simulink library "halout"  (R2021b)
settings: Solver=VariableStepAuto  StartTime=0.0  StopTime=10.0  RelTol=1e-3
undefined symbols (not defined in the file): C_TASK_5MS_S, FALSE, KHAL_CAN1FD1APS3E2E_flg, KHAL_CAN1FD1APS3TxReq_flg, KHAL_CAN1FD1VCU2E2E_flg, KHAL_CAN1FD1VCU2TxReq_flg, KHAL_CAN1FD1VCU3E2E_flg, KHAL_CAN1FD1VCU3TxReq_flg, KHAL_CAN1TxReq_flg, KHAL_CAN1VMCFCM1E2E_flg, KHAL_CAN1VMCFCM1TxReq_flg, KHAL_CAN2TxReq_flg, KHAL_CAN3FD3VCU1toNIDECTxReq_flg, KHAL_CAN3FD3VCU1TxReq_flg, KHAL_CAN3FD3VCU2E2E_flg, KHAL_CAN3FD3VCU2toNIDECE2E_flg, KHAL_CAN3FD3VCU2toNIDECTxReq_flg, KHAL_CAN3FD3VCU2TxReq_flg, KHAL_CAN3TxReq_flg, KHAL_CAN4FD4CE1000E2E_flg, KHAL_CAN4FD4CE1000TxReq_flg, KHAL_CAN4TxReq_flg, KHAL_CAN5TxReq_flg, KHAL_CAN6FD6APS3E2E_flg, KHAL_CAN6FD6APS3TxReq_flg, KHAL_CAN6FD6VCU2E2E_flg, KHAL_CAN6FD6VCU2TxReq_flg, KHAL_CAN6TxReq_flg, ONE_INT, TRUE, ZERO_INT
libraries: FVT_lib x549, simulink x244
(part 7 of 27)

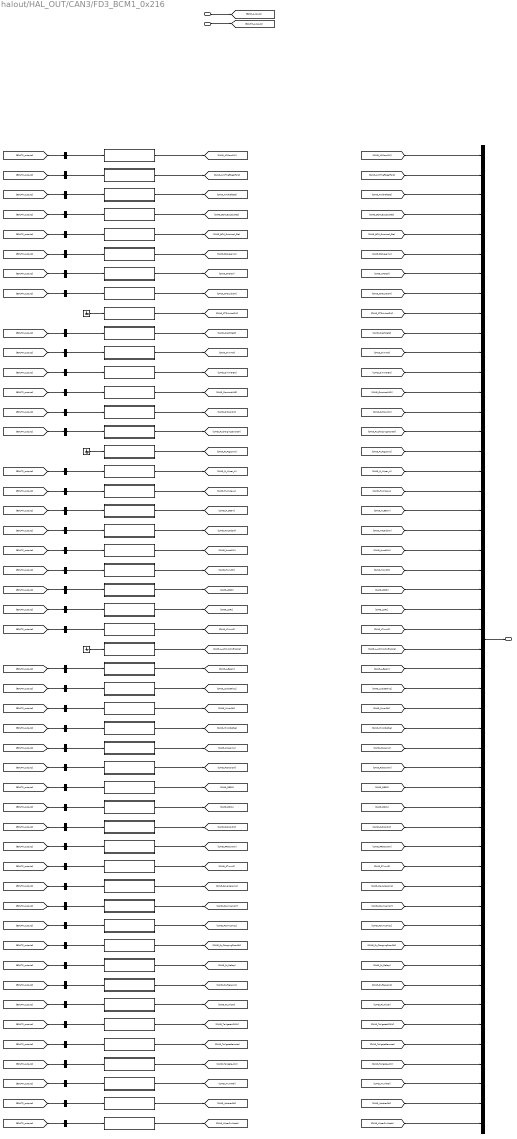
== system halout/HAL_OUT/CAN3/FD3_BCM1_0x216 ==
  BSCP_outputs : Inport  OutDataTypeStr=Bus: BSCP_outputs
  BOUTP_outputs : Inport  Port=2  OutDataTypeStr=Bus: BOUTP_outputs
  AllDoorSW : Subsystem
  AntiTheftSeatFold : Subsystem
  AntitheftSta : Subsystem
  BCMBuzzerReq : Subsystem
  BCMDoorLockSta : Subsystem
  BrakeLamp : Subsystem
  CTDCtrl : Subsystem
  CTDLockSW : Subsystem
  CTDUnlockSW : Subsystem
  CrashDetd : Subsystem
  Dimmer : Subsystem
  DimmerEN : Subsystem
  DoorLockIND : Subsystem
  DrDoorSW : Subsystem
  FrChargingDoorCtrl : Subsystem
  FrFogLamp : Subsystem
  FrWiperH : Subsystem
  FrWiperL : Subsystem
  Ground : Ground
  Ground1 : Ground
  Ground2 : Ground
  HBeam : Subsystem
  HazardSW : Subsystem
  HoodSW : Subsystem
  HornCtrl : Subsystem
  LAPMWdwEnable : Subsystem
  LBSD : Subsystem
  LBeam : Subsystem
  LDRL : Subsystem
  LTurnLP : Subsystem
  LockSetting : Subsystem
  MirrorCtrl : Subsystem
  MirrorDefog : Subsystem
  PosLamp : Subsystem
  PsDoorSW : Subsystem
  RBSD : Subsystem
  RDRL : Subsystem
  RLDoorSW : Subsystem
  RRDoorSW : Subsystem
  RTurnLP : Subsystem
  ReverseLamp : Subsystem
  RoomLampH : Subsystem
  RoomLampL : Subsystem
  RrChargingDoorCtrl : Subsystem
  RrDefog : Subsystem
  RrFogLamp : Subsystem
  RrWiper : Subsystem
  TailgateHDSW : Subsystem
  TailgateRemote : Subsystem
  TailgateSW : Subsystem
  TrunkRel : Subsystem
  WasherCtrl : Subsystem
  WiperFixMode : Subsystem
  bus_creator : BusCreator  Inputs=50  OutDataTypeStr=Bus: DT_CAN3_SG_FD3_BCM1  NonVirtualBus=on
  bus_selector : BusSelector  OutputSignals=VOUTP_AllDoorSW_flg
  bus_selector1 : BusSelector  OutputSignals=VOUTP_AntitheftSeatFlod_flg
  bus_selector10 : BusSelector  OutputSignals=VOUTP_DimmerEN_flg
  bus_selector11 : BusSelector  OutputSignals=VOUTP_DoorLockIND_flg
  bus_selector12 : BusSelector  OutputSignals=VOUTP_DrDoorSW_flg
  bus_selector13 : BusSelector  OutputSignals=VOUTP_FrChargingDoorCtrl_enum
  bus_selector14 : BusSelector  OutputSignals=VOUTP_FrWiperH_flg
  bus_selector15 : BusSelector  OutputSignals=VOUTP_FrWiperL_flg
  bus_selector16 : BusSelector  OutputSignals=VOUTP_HBeam_flg
  bus_selector17 : BusSelector  OutputSignals=VOUTP_HazardSW_flg
  bus_selector18 : BusSelector  OutputSignals=VOUTP_HoodSW_flg
  bus_selector19 : BusSelector  OutputSignals=VOUTP_HornCtrl_flg
  bus_selector2 : BusSelector  OutputSignals=VOUTP_AntitheftSta_enum
  bus_selector20 : BusSelector  OutputSignals=VOUTP_LBSD_flg
  bus_selector21 : BusSelector  OutputSignals=VOUTP_LDRL_flg
  bus_selector22 : BusSelector  OutputSignals=VOUTP_LTurnLP_flg
  bus_selector23 : BusSelector  OutputSignals=VOUTP_LBeam_flg
  bus_selector24 : BusSelector  OutputSignals=VOUTP_LockSetting_flg
  bus_selector25 : BusSelector  OutputSignals=VOUTP_MirrorCtrl_enum
  bus_selector26 : BusSelector  OutputSignals=VOUTP_MirrorDefog_flg
  bus_selector27 : BusSelector  OutputSignals=VOUTP_PosLamp_flg
  bus_selector28 : BusSelector  OutputSignals=VOUTP_PsDoorSW_flg
  bus_selector29 : BusSelector  OutputSignals=VOUTP_RBSD_flg
  bus_selector3 : BusSelector  OutputSignals=VOUTP_BCMBuzzerReq_flg
  bus_selector30 : BusSelector  OutputSignals=VOUTP_RDRL_flg
  bus_selector31 : BusSelector  OutputSignals=VOUTP_RLDoorSW_flg
  bus_selector32 : BusSelector  OutputSignals=VOUTP_RRDoorSW_flg
  bus_selector33 : BusSelector  OutputSignals=VOUTP_RTurnLP_flg
  bus_selector34 : BusSelector  OutputSignals=VOUTP_ReverseLamp_flg
  bus_selector35 : BusSelector  OutputSignals=VOUTP_RoomLampH_flg
  bus_selector36 : BusSelector  OutputSignals=VOUTP_RoomLampL_flg
  bus_selector37 : BusSelector  OutputSignals=VOUTP_RrChargingDoorCtrl_enum
  bus_selector38 : BusSelector  OutputSignals=VOUTP_RrDefog_flg
  bus_selector39 : BusSelector  OutputSignals=VOUTP_RrFogLamp_flg
  bus_selector4 : BusSelector  OutputSignals=VOUTP_BCMDoorLockSta_flg
  bus_selector40 : BusSelector  OutputSignals=VOUTP_RrWiper_flg
  bus_selector41 : BusSelector  OutputSignals=VOUTP_TailgateHDSW_flg
  bus_selector42 : BusSelector  OutputSignals=VOUTP_TailgateRemote_enum
  bus_selector43 : BusSelector  OutputSignals=VOUTP_TailgateSW_flg
  bus_selector44 : BusSelector  OutputSignals=VOUTP_TrunkRel_flg
  bus_selector45 : BusSelector  OutputSignals=VOUTP_WasherCtrl_enum
  bus_selector46 : BusSelector  OutputSignals=VOUTP_WiperFixMode_flg
  bus_selector5 : BusSelector  OutputSignals=VOUTP_BrakeLamp_flg
  bus_selector6 : BusSelector  OutputSignals=VOUTP_CTDCtrl_enum
  bus_selector7 : BusSelector  OutputSignals=VOUTP_CTDLockSW_flg
  bus_selector8 : BusSelector  OutputSignals=VOUTP_CrashDetd_flg
  bus_selector9 : BusSelector  OutputSignals=VOUTP_Dimmer_pct
  FD3_BCM1 : Outport
  wires:
  BSCP_outputs/1 -> [BSCP_outputs]
  BOUTP_outputs/1 -> [BOUTP_outputs]
  [CAN3_AllDoorSW] -> bus_creator/1  "CAN3_AllDoorSW"
  [CAN3_AntiTheftSeatFold] -> bus_creator/2  "CAN3_AntiTheftSeatFold"
  [CAN3_AntitheftSta] -> bus_creator/3  "CAN3_AntitheftSta"
  [CAN3_BCM_Buzzer_Req] -> bus_creator/4  "CAN3_BCM_Buzzer_Req"
  [CAN3_BCM_DoorLock_Sta] -> bus_creator/5  "CAN3_BCM_DoorLock_Sta"
  [CAN3_BrakeLamp] -> bus_creator/6  "CAN3_BrakeLamp"
  [CAN3_CTDCtrl] -> bus_creator/7  "CAN3_CTDCtrl"
  [CAN3_CTDLockSW] -> bus_creator/8  "CAN3_CTDLockSW"
  [CAN3_CTDUnlockSW] -> bus_creator/9  "CAN3_CTDUnlockSW"
  [CAN3_CrashDetd] -> bus_creator/10  "CAN3_CrashDetd"
  [CAN3_Dimmer] -> bus_creator/11  "CAN3_Dimmer"
  [CAN3_DimmerEN] -> bus_creator/12  "CAN3_DimmerEN"
  [CAN3_DoorLockIND] -> bus_creator/13  "CAN3_DoorLockIND"
  [CAN3_DrDoorSW] -> bus_creator/14  "CAN3_DrDoorSW"
  [CAN3_Fr_ChargingDoorCtrl] -> bus_creator/15  "CAN3_Fr_ChargingDoorCtrl"
  [CAN3_Fr_FogLamp] -> bus_creator/16  "CAN3_Fr_FogLamp"
  [CAN3_Fr_Wiper_H] -> bus_creator/17  "CAN3_Fr_Wiper_H"
  [CAN3_Fr_Wiper_L] -> bus_creator/18  "CAN3_Fr_Wiper_L"
  [CAN3_H_Beam] -> bus_creator/19  "CAN3_H_Beam"
  [CAN3_HazardSW] -> bus_creator/20  "CAN3_HazardSW"
  [CAN3_HoodSW] -> bus_creator/21  "CAN3_HoodSW"
  [CAN3_HornCtrl] -> bus_creator/22  "CAN3_HornCtrl"
  [CAN3_LBSD] -> bus_creator/23  "CAN3_LBSD"
  [CAN3_LDRL] -> bus_creator/24  "CAN3_LDRL"
  [CAN3_LTurnLP] -> bus_creator/25  "CAN3_LTurnLP"
  [CAN3_L_APM_WdwEnable] -> bus_creator/26  "CAN3_L_APM_WdwEnable"
  [CAN3_L_Beam] -> bus_creator/27  "CAN3_L_Beam"
  [CAN3_LockSetting] -> bus_creator/28  "CAN3_LockSetting"
  [CAN3_MirrorCtrl] -> bus_creator/29  "CAN3_MirrorCtrl"
  [CAN3_MirrorDefog] -> bus_creator/30  "CAN3_MirrorDefog"
  [CAN3_PosLamp] -> bus_creator/31  "CAN3_PosLamp"
  [CAN3_PsDoorSW] -> bus_creator/32  "CAN3_PsDoorSW"
  [CAN3_RBSD] -> bus_creator/33  "CAN3_RBSD"
  [CAN3_RDRL] -> bus_creator/34  "CAN3_RDRL"
  [CAN3_RLDoorSW] -> bus_creator/35  "CAN3_RLDoorSW"
  [CAN3_RRDoorSW] -> bus_creator/36  "CAN3_RRDoorSW"
  [CAN3_RTurnLP] -> bus_creator/37  "CAN3_RTurnLP"
  [CAN3_ReverseLamp] -> bus_creator/38  "CAN3_ReverseLamp"
  [CAN3_RoomLampH] -> bus_creator/39  "CAN3_RoomLampH"
  [CAN3_RoomLampL] -> bus_creator/40  "CAN3_RoomLampL"
  [CAN3_Rr_ChargingDoorCtrl] -> bus_creator/41  "CAN3_Rr_ChargingDoorCtrl"
  [CAN3_Rr_Defog] -> bus_creator/42  "CAN3_Rr_Defog"
  [CAN3_Rr_FogLamp] -> bus_creator/43  "CAN3_Rr_FogLamp"
  [CAN3_Rr_Wiper] -> bus_creator/44  "CAN3_Rr_Wiper"
  [CAN3_TailgateHDSW] -> bus_creator/45  "CAN3_TailgateHDSW"
  [CAN3_TailgateRemote] -> bus_creator/46  "CAN3_TailgateRemote"
  [CAN3_Tailgate_SW] -> bus_creator/47  "CAN3_Tailgate_SW"
  [CAN3_TrunkRel] -> bus_creator/48  "CAN3_TrunkRel"
  [CAN3_WasherCtrl] -> bus_creator/49  "CAN3_WasherCtrl"
  [CAN3_WiperFixMode] -> bus_creator/50  "CAN3_WiperFixMode"
  bus_creator/1 -> FD3_BCM1/1
  AllDoorSW/1(CAN3_AllDoorSW) -> [CAN3_AllDoorSW]
  AntiTheftSeatFold/1(CAN3_AntiTheftSeatFold) -> [CAN3_AntiTheftSeatFold]
  AntitheftSta/1(CAN3_AntitheftSta) -> [CAN3_AntitheftSta]
  BCMBuzzerReq/1(CAN3_BCM_Buzzer_Req) -> [CAN3_BCM_Buzzer_Req]
  BCMDoorLockSta/1(CAN3_BCM_DoorLock_Sta) -> [CAN3_BCM_DoorLock_Sta]
  BrakeLamp/1(CAN3_BrakeLamp) -> [CAN3_BrakeLamp]
  CTDCtrl/1(CAN3_CTDCtrl) -> [CAN3_CTDCtrl]
  CTDLockSW/1(CAN3_CTDLockSW) -> [CAN3_CTDLockSW]
  CTDUnlockSW/1(CAN3_CTDUnlockSW) -> [CAN3_CTDUnlockSW]
  CrashDetd/1(CAN3_CrashDetd) -> [CAN3_CrashDetd]
  Dimmer/1(CAN3_Dimmer) -> [CAN3_Dimmer]
  DimmerEN/1(CAN3_DimmerEN) -> [CAN3_DimmerEN]
  DoorLockIND/1(CAN3_DoorLockIND) -> [CAN3_DoorLockIND]
  DrDoorSW/1(CAN3_DrDoorSW) -> [CAN3_DrDoorSW]
  FrChargingDoorCtrl/1(CAN3_Fr_ChargingDoorCtrl) -> [CAN3_Fr_ChargingDoorCtrl]
  FrFogLamp/1(CAN3_Fr_FogLamp) -> [CAN3_Fr_FogLamp]
  FrWiperH/1(CAN3_Fr_Wiper_H) -> [CAN3_Fr_Wiper_H]
  FrWiperL/1(CAN3_Fr_Wiper_L) -> [CAN3_Fr_Wiper_L]
  HBeam/1(CAN3_H_Beam) -> [CAN3_H_Beam]
  HazardSW/1(CAN3_HazardSW) -> [CAN3_HazardSW]
  HoodSW/1(CAN3_HoodSW) -> [CAN3_HoodSW]
  HornCtrl/1(CAN3_HornCtrl) -> [CAN3_HornCtrl]
  LBSD/1(CAN3_LBSD) -> [CAN3_LBSD]
  LDRL/1(CAN3_LDRL) -> [CAN3_LDRL]
  LTurnLP/1(CAN3_LTurnLP) -> [CAN3_LTurnLP]
  LAPMWdwEnable/1(CAN3_L_APM_WdwEnable) -> [CAN3_L_APM_WdwEnable]
  LBeam/1(CAN3_L_Beam) -> [CAN3_L_Beam]
  LockSetting/1(CAN3_LockSetting) -> [CAN3_LockSetting]
  MirrorCtrl/1(CAN3_MirrorCtrl) -> [CAN3_MirrorCtrl]
  MirrorDefog/1(CAN3_MirrorDefog) -> [CAN3_MirrorDefog]
  PosLamp/1(CAN3_PosLamp) -> [CAN3_PosLamp]
  PsDoorSW/1(CAN3_PsDoorSW) -> [CAN3_PsDoorSW]
  RBSD/1(CAN3_RBSD) -> [CAN3_RBSD]
  RDRL/1(CAN3_RDRL) -> [CAN3_RDRL]
  RLDoorSW/1(CAN3_RLDoorSW) -> [CAN3_RLDoorSW]
  RRDoorSW/1(CAN3_RRDoorSW) -> [CAN3_RRDoorSW]
  RTurnLP/1(CAN3_RTurnLP) -> [CAN3_RTurnLP]
  ReverseLamp/1(CAN3_ReverseLamp) -> [CAN3_ReverseLamp]
  RoomLampH/1(CAN3_RoomLampH) -> [CAN3_RoomLampH]
  RoomLampL/1(CAN3_RoomLampL) -> [CAN3_RoomLampL]
  RrChargingDoorCtrl/1(CAN3_Rr_ChargingDoorCtrl) -> [CAN3_Rr_ChargingDoorCtrl]
  RrDefog/1(CAN3_Rr_Defog) -> [CAN3_Rr_Defog]
  RrFogLamp/1(CAN3_Rr_FogLamp) -> [CAN3_Rr_FogLamp]
  RrWiper/1(CAN3_Rr_Wiper) -> [CAN3_Rr_Wiper]
  TailgateHDSW/1(CAN3_TailgateHDSW) -> [CAN3_TailgateHDSW]
  TailgateRemote/1(CAN3_TailgateRemote) -> [CAN3_TailgateRemote]
  TailgateSW/1(CAN3_Tailgate_SW) -> [CAN3_Tailgate_SW]
  TrunkRel/1(CAN3_TrunkRel) -> [CAN3_TrunkRel]
  WasherCtrl/1(CAN3_WasherCtrl) -> [CAN3_WasherCtrl]
  WiperFixMode/1(CAN3_WiperFixMode) -> [CAN3_WiperFixMode]
  bus_selector/1 -> AllDoorSW/1(AllDoorSW)  "<VOUTP_AllDoorSW_flg>"
  [BOUTP_outputs] -> bus_selector/1
  bus_selector1/1 -> AntiTheftSeatFold/1(AntiTheftSeatFold)  "<VOUTP_AntitheftSeatFlod_flg>"
  [BOUTP_outputs] -> bus_selector1/1
  bus_selector2/1 -> AntitheftSta/1(AntitheftSta)  "<VOUTP_AntitheftSta_enum>"
  [BOUTP_outputs] -> bus_selector2/1
  bus_selector3/1 -> BCMBuzzerReq/1(BCMBuzzerReq)  "<VOUTP_BCMBuzzerReq_flg>"
  [BOUTP_outputs] -> bus_selector3/1
  bus_selector4/1 -> BCMDoorLockSta/1(BCMDoorLockSta)  "<VOUTP_BCMDoorLockSta_flg>"
  [BOUTP_outputs] -> bus_selector4/1
  bus_selector5/1 -> BrakeLamp/1(BrakeLamp)  "<VOUTP_BrakeLamp_flg>"
  [BOUTP_outputs] -> bus_selector5/1
  bus_selector6/1 -> CTDCtrl/1(CTDCtrl)  "<VOUTP_CTDCtrl_enum>"
  [BOUTP_outputs] -> bus_selector6/1
  bus_selector7/1 -> CTDLockSW/1(CTDLockSW)  "<VOUTP_CTDLockSW_flg>"
  [BOUTP_outputs] -> bus_selector7/1
  Ground/1 -> CTDUnlockSW/1(CTDUnlockSW)
  bus_selector8/1 -> CrashDetd/1(CrashDetd)  "<VOUTP_CrashDetd_flg>"
  [BOUTP_outputs] -> bus_selector8/1
  bus_selector9/1 -> Dimmer/1(Dimmer)  "<VOUTP_Dimmer_pct>"
  [BOUTP_outputs] -> bus_selector9/1
  bus_selector10/1 -> DimmerEN/1(DimmerEN)  "<VOUTP_DimmerEN_flg>"
  [BOUTP_outputs] -> bus_selector10/1
  bus_selector11/1 -> DoorLockIND/1(DoorLockIND)  "<VOUTP_DoorLockIND_flg>"
  [BOUTP_outputs] -> bus_selector11/1
  bus_selector12/1 -> DrDoorSW/1(DrDoorSW)  "<VOUTP_DrDoorSW_flg>"
  [BOUTP_outputs] -> bus_selector12/1
  bus_selector13/1 -> FrChargingDoorCtrl/1(FrChargingDoorCtrl)  "<VOUTP_FrChargingDoorCtrl_enum>"
  [BOUTP_outputs] -> bus_selector13/1
  Ground1/1 -> FrFogLamp/1(FrFogLamp)
  bus_selector14/1 -> FrWiperH/1(FrWiperH)  "<VOUTP_FrWiperH_flg>"
  [BOUTP_outputs] -> bus_selector14/1
  bus_selector15/1 -> FrWiperL/1(FrWiperL)  "<VOUTP_FrWiperL_flg>"
  [BOUTP_outputs] -> bus_selector15/1
  bus_selector16/1 -> HBeam/1(HBeam)  "<VOUTP_HBeam_flg>"
  [BOUTP_outputs] -> bus_selector16/1
  bus_selector17/1 -> HazardSW/1(HazardSW)  "<VOUTP_HazardSW_flg>"
  [BOUTP_outputs] -> bus_selector17/1
  bus_selector18/1 -> HoodSW/1(HoodSW)  "<VOUTP_HoodSW_flg>"
  [BOUTP_outputs] -> bus_selector18/1
  bus_selector19/1 -> HornCtrl/1(HornCtrl)  "<VOUTP_HornCtrl_flg>"
  [BOUTP_outputs] -> bus_selector19/1
  bus_selector20/1 -> LBSD/1(LBSD)  "<VOUTP_LBSD_flg>"
  [BOUTP_outputs] -> bus_selector20/1
  bus_selector21/1 -> LDRL/1(LDRL)  "<VOUTP_LDRL_flg>"
  [BOUTP_outputs] -> bus_selector21/1
  bus_selector22/1 -> LTurnLP/1(LTurnLP)  "<VOUTP_LTurnLP_flg>"
  [BOUTP_outputs] -> bus_selector22/1
  Ground2/1 -> LAPMWdwEnable/1(LAPMWdwEnable)
  bus_selector23/1 -> LBeam/1(LBeam)  "<VOUTP_LBeam_flg>"
  [BOUTP_outputs] -> bus_selector23/1
  bus_selector24/1 -> LockSetting/1(LockSetting)  "<VOUTP_LockSetting_flg>"
  [BOUTP_outputs] -> bus_selector24/1
  bus_selector25/1 -> MirrorCtrl/1(MirrorCtrl)  "<VOUTP_MirrorCtrl_enum>"
  [BOUTP_outputs] -> bus_selector25/1
  bus_selector26/1 -> MirrorDefog/1(MirrorDefog)  "<VOUTP_MirrorDefog_flg>"
  [BOUTP_outputs] -> bus_selector26/1
  bus_selector27/1 -> PosLamp/1(PosLamp)  "<VOUTP_PosLamp_flg>"
  [BOUTP_outputs] -> bus_selector27/1
  bus_selector28/1 -> PsDoorSW/1(PsDoorSW)  "<VOUTP_PsDoorSW_flg>"
  [BOUTP_outputs] -> bus_selector28/1
  bus_selector29/1 -> RBSD/1(RBSD)  "<VOUTP_RBSD_flg>"
  [BOUTP_outputs] -> bus_selector29/1
  bus_selector30/1 -> RDRL/1(RDRL)  "<VOUTP_RDRL_flg>"
  [BOUTP_outputs] -> bus_selector30/1
  bus_selector31/1 -> RLDoorSW/1(RLDoorSW)  "<VOUTP_RLDoorSW_flg>"
  [BOUTP_outputs] -> bus_selector31/1
  bus_selector32/1 -> RRDoorSW/1(RRDoorSW)  "<VOUTP_RRDoorSW_flg>"
  [BOUTP_outputs] -> bus_selector32/1
  bus_selector33/1 -> RTurnLP/1(RTurnLP)  "<VOUTP_RTurnLP_flg>"
  [BOUTP_outputs] -> bus_selector33/1
  bus_selector34/1 -> ReverseLamp/1(ReverseLamp)  "<VOUTP_ReverseLamp_flg>"
  [BOUTP_outputs] -> bus_selector34/1
  bus_selector35/1 -> RoomLampH/1(RoomLampH)  "<VOUTP_RoomLampH_flg>"
  [BOUTP_outputs] -> bus_selector35/1
  bus_selector36/1 -> RoomLampL/1(RoomLampL)  "<VOUTP_RoomLampL_flg>"
  [BOUTP_outputs] -> bus_selector36/1
  bus_selector37/1 -> RrChargingDoorCtrl/1(RrChargingDoorCtrl)  "<VOUTP_RrChargingDoorCtrl_enum>"
  [BOUTP_outputs] -> bus_selector37/1
  bus_selector38/1 -> RrDefog/1(RrDefog)  "<VOUTP_RrDefog_flg>"
  [BOUTP_outputs] -> bus_selector38/1
  bus_selector39/1 -> RrFogLamp/1(RrFogLamp)  "<VOUTP_RrFogLamp_flg>"
  [BOUTP_outputs] -> bus_selector39/1
  bus_selector40/1 -> RrWiper/1(RrWiper)  "<VOUTP_RrWiper_flg>"
  [BOUTP_outputs] -> bus_selector40/1
  bus_selector41/1 -> TailgateHDSW/1(TailgateHDSW)  "<VOUTP_TailgateHDSW_flg>"
  [BOUTP_outputs] -> bus_selector41/1
  bus_selector42/1 -> TailgateRemote/1(TailgateRemote)  "<VOUTP_TailgateRemote_enum>"
  [BOUTP_outputs] -> bus_selector42/1
  bus_selector43/1 -> TailgateSW/1(TailgateSW)  "<VOUTP_TailgateSW_flg>"
  [BOUTP_outputs] -> bus_selector43/1
  bus_selector44/1 -> TrunkRel/1(TrunkRel)  "<VOUTP_TrunkRel_flg>"
  [BOUTP_outputs] -> bus_selector44/1
  bus_selector45/1 -> WasherCtrl/1(WasherCtrl)  "<VOUTP_WasherCtrl_enum>"
  [BOUTP_outputs] -> bus_selector45/1
  bus_selector46/1 -> WiperFixMode/1(WiperFixMode)  "<VOUTP_WiperFixMode_flg>"
  [BOUTP_outputs] -> bus_selector46/1

== system halout/HAL_OUT/CAN3/FD3_THCM1_0x182 ==
  BSCP_outputs : Inport  OutDataTypeStr=Bus: BSCP_outputs
  BOUTP_outputs : Inport  Port=2  OutDataTypeStr=Bus: BOUTP_outputs
  BatteryMode : Subsystem
  CCUACLampSts : Subsystem
  CCUACMaxLampSts : Subsystem
  CCUAutoLampSts : Subsystem
  CCUAutoMidLampSts : Subsystem
  CCUDispalyRequest : Subsystem
  CCUEcoSts : Subsystem
  CCUFrtOnOffLampSts : Subsystem
  CCUHEATMaxLampSts : Subsystem
  CCURrOnOffLampSts : Subsystem
  CCUSyncLampSts : Subsystem
  CabinMode : Subsystem
  EDriveMode : Subsystem
  FDAGSCmd : Subsystem
  FDRecyAutoCmd : Subsystem
  FrCoolantflow : Subsystem
  FrCoolanttemp : Subsystem
  Ground{,1..16} (17 alike) : Ground
  HPThermalRecoveryReq : Subsystem
  RrCoolantflow : Subsystem
  RrCoolanttemp : Subsystem
  bus_creator : BusCreator  Inputs=37  OutDataTypeStr=Bus: DT_CAN3_SG_FD3_THCM1  NonVirtualBus=on
  bus_selector : BusSelector  OutputSignals=VOUTP_BatteryMode_enum
  bus_selector1 : BusSelector  OutputSignals=VOUTP_CCUACLampSts_flg
  bus_selector10 : BusSelector  OutputSignals=VOUTP_sigAmbAirT_C
  bus_selector11 : BusSelector  OutputSignals=VOUTP_sigCbnAirT_C
  bus_selector12 : BusSelector  OutputSignals=VOUTP_sigCbnSolarLeft_W
  bus_selector13 : BusSelector  OutputSignals=VOUTP_sigCbnSolarRight_W
  bus_selector14 : BusSelector  OutputSignals=VOUTP_sigClntTHvBattOut_C
  bus_selector15 : BusSelector  OutputSignals=VOUTP_sigDfrstSt_flg
  bus_selector16 : BusSelector  OutputSignals=VOUTP_sigRecircSt_flg
  bus_selector17 : BusSelector  OutputSignals=VOUTP_sigSetTempZon1St_C
  bus_selector18 : BusSelector  OutputSignals=VOUTP_sigSetTempZon2St_C
  bus_selector19 : BusSelector  OutputSignals=VOUTP_sigWindDirZon1St_enum
  bus_selector2 : BusSelector  OutputSignals=VOUTP_CCUACMaxLampSts_flg
  bus_selector3 : BusSelector  OutputSignals=VOUTP_CCUAutoLampSts_flg
  bus_selector4 : BusSelector  OutputSignals=VOUTP_CCUSyncLampSts_flg
  bus_selector5 : BusSelector  OutputSignals=VOUTP_CabinMode_enum
  bus_selector6 : BusSelector  OutputSignals=VOUTP_EDriveMode_enum
  bus_selector7 : BusSelector  OutputSignals=VOUTP_FDAGSCmd_enum
  bus_selector8 : BusSelector  OutputSignals=VOUTP_FDRecyAutoCmd_enum
  bus_selector9 : BusSelector  OutputSignals=VOUTP_sigAirIntenZon1St_enum
  sigAirIntenZon1St : Subsystem
  sigAirIntenZon3St : Subsystem
  sigAmbAirT : Subsystem
  sigCbnAirT : Subsystem
  sigCbnPTCPwrAct : Subsystem
  sigCbnSolarLeft : Subsystem
  sigCbnSolarRight : Subsystem
  sigClmtCmprPwrAct : Subsystem
  sigClntTHvBattOut : Subsystem
  sigDfrstSt : Subsystem
  sigHvacSt : Subsystem
  sigRecircSt : Subsystem
  sigSetTempZon1St : Subsystem
  sigSetTempZon2St : Subsystem
  sigSetTempZon3St : Subsystem
  sigWindDirZon1St : Subsystem
  sigWindDirZon3St : Subsystem
  FD3_THCM1 : Outport
  wires:
  BSCP_outputs/1 -> [BSCP_outputs]
  BOUTP_outputs/1 -> [BOUTP_outputs]
  [CAN3_BatteryMode] -> bus_creator/1  "CAN3_BatteryMode"
  [CAN3_CCU_ACLampSts] -> bus_creator/2  "CAN3_CCU_ACLampSts"
  [CAN3_CCU_ACMaxLampSts] -> bus_creator/3  "CAN3_CCU_ACMaxLampSts"
  [CAN3_CCU_AutoLampSts] -> bus_creator/4  "CAN3_CCU_AutoLampSts"
  [CAN3_CCU_AutoMidLampSts] -> bus_creator/5  "CAN3_CCU_AutoMidLampSts"
  [CAN3_CCU_Dispaly_Request] -> bus_creator/6  "CAN3_CCU_Dispaly_Request"
  [CAN3_CCU_EcoSts] -> bus_creator/7  "CAN3_CCU_EcoSts"
  [CAN3_CCU_FrtOnOffLampSts] -> bus_creator/8  "CAN3_CCU_FrtOnOffLampSts"
  [CAN3_CCU_HEATMaxLampSts] -> bus_creator/9  "CAN3_CCU_HEATMaxLampSts"
  [CAN3_CCU_RrOnOffLampSts] -> bus_creator/10  "CAN3_CCU_RrOnOffLampSts"
  [CAN3_CCU_SyncLampSts] -> bus_creator/11  "CAN3_CCU_SyncLampSts"
  [CAN3_CabinMode] -> bus_creator/12  "CAN3_CabinMode"
  [CAN3_EDriveMode] -> bus_creator/13  "CAN3_EDriveMode"
  [CAN3_FD_AGS_Cmd] -> bus_creator/14  "CAN3_FD_AGS_Cmd"
  [CAN3_FD_RecyAuto_Cmd] -> bus_creator/15  "CAN3_FD_RecyAuto_Cmd"
  [CAN3_Fr_Coolantflow] -> bus_creator/16  "CAN3_Fr_Coolantflow"
  [CAN3_Fr_Coolanttemp] -> bus_creator/17  "CAN3_Fr_Coolanttemp"
  [CAN3_HPThermalRecoveryReq] -> bus_creator/18  "CAN3_HPThermalRecoveryReq"
  [CAN3_Rr_Coolantflow] -> bus_creator/19  "CAN3_Rr_Coolantflow"
  [CAN3_Rr_Coolanttemp] -> bus_creator/20  "CAN3_Rr_Coolanttemp"
  [CAN3_sigAirIntenZon1St] -> bus_creator/21  "CAN3_sigAirIntenZon1St"
  [CAN3_sigAirIntenZon3St] -> bus_creator/22  "CAN3_sigAirIntenZon3St"
  [CAN3_sigAmbAirT] -> bus_creator/23  "CAN3_sigAmbAirT"
  [CAN3_sigCbnAirT] -> bus_creator/24  "CAN3_sigCbnAirT"
  [CAN3_sigCbnPTCPwrAct] -> bus_creator/25  "CAN3_sigCbnPTCPwrAct"
  [CAN3_sigCbnSolarLeft] -> bus_creator/26  "CAN3_sigCbnSolarLeft"
  [CAN3_sigCbnSolarRight] -> bus_creator/27  "CAN3_sigCbnSolarRight"
  [CAN3_sigClmtCmprPwrAct] -> bus_creator/28  "CAN3_sigClmtCmprPwrAct"
  [CAN3_sigClntTHvBattOut] -> bus_creator/29  "CAN3_sigClntTHvBattOut"
  [CAN3_sigDfrstSt] -> bus_creator/30  "CAN3_sigDfrstSt"
  [CAN3_sigHvacSt] -> bus_creator/31  "CAN3_sigHvacSt"
  [CAN3_sigRecircSt] -> bus_creator/32  "CAN3_sigRecircSt"
  [CAN3_sigSetTempZon1St] -> bus_creator/33  "CAN3_sigSetTempZon1St"
  [CAN3_sigSetTempZon2St] -> bus_creator/34  "CAN3_sigSetTempZon2St"
  [CAN3_sigSetTempZon3St] -> bus_creator/35  "CAN3_sigSetTempZon3St"
  [CAN3_sigWindDirZon1St] -> bus_creator/36  "CAN3_sigWindDirZon1St"
  [CAN3_sigWindDirZon3St] -> bus_creator/37  "CAN3_sigWindDirZon3St"
  bus_creator/1 -> FD3_THCM1/1
  BatteryMode/1(CAN3_BatteryMode) -> [CAN3_BatteryMode]
  CCUACLampSts/1(CAN3_CCU_ACLampSts) -> [CAN3_CCU_ACLampSts]
  CCUACMaxLampSts/1(CAN3_CCU_ACMaxLampSts) -> [CAN3_CCU_ACMaxLampSts]
  CCUAutoLampSts/1(CAN3_CCU_AutoLampSts) -> [CAN3_CCU_AutoLampSts]
  CCUAutoMidLampSts/1(CAN3_CCU_AutoMidLampSts) -> [CAN3_CCU_AutoMidLampSts]
  CCUDispalyRequest/1(CAN3_CCU_Dispaly_Request) -> [CAN3_CCU_Dispaly_Request]
  CCUEcoSts/1(CAN3_CCU_EcoSts) -> [CAN3_CCU_EcoSts]
  CCUFrtOnOffLampSts/1(CAN3_CCU_FrtOnOffLampSts) -> [CAN3_CCU_FrtOnOffLampSts]
  CCUHEATMaxLampSts/1(CAN3_CCU_HEATMaxLampSts) -> [CAN3_CCU_HEATMaxLampSts]
  CCURrOnOffLampSts/1(CAN3_CCU_RrOnOffLampSts) -> [CAN3_CCU_RrOnOffLampSts]
  CCUSyncLampSts/1(CAN3_CCU_SyncLampSts) -> [CAN3_CCU_SyncLampSts]
  CabinMode/1(CAN3_CabinMode) -> [CAN3_CabinMode]
  EDriveMode/1(CAN3_EDriveMode) -> [CAN3_EDriveMode]
  FDAGSCmd/1(CAN3_FD_AGS_Cmd) -> [CAN3_FD_AGS_Cmd]
  FDRecyAutoCmd/1(CAN3_FD_RecyAuto_Cmd) -> [CAN3_FD_RecyAuto_Cmd]
  FrCoolantflow/1(CAN3_Fr_Coolantflow) -> [CAN3_Fr_Coolantflow]
  FrCoolanttemp/1(CAN3_Fr_Coolanttemp) -> [CAN3_Fr_Coolanttemp]
  HPThermalRecoveryReq/1(CAN3_HPThermalRecoveryReq) -> [CAN3_HPThermalRecoveryReq]
  RrCoolantflow/1(CAN3_Rr_Coolantflow) -> [CAN3_Rr_Coolantflow]
  RrCoolanttemp/1(CAN3_Rr_Coolanttemp) -> [CAN3_Rr_Coolanttemp]
  sigAirIntenZon1St/1(CAN3_sigAirIntenZon1St) -> [CAN3_sigAirIntenZon1St]
  sigAirIntenZon3St/1(CAN3_sigAirIntenZon3St) -> [CAN3_sigAirIntenZon3St]
  sigAmbAirT/1(CAN3_sigAmbAirT) -> [CAN3_sigAmbAirT]
  sigCbnAirT/1(CAN3_sigCbnAirT) -> [CAN3_sigCbnAirT]
  sigCbnPTCPwrAct/1(CAN3_sigCbnPTCPwrAct) -> [CAN3_sigCbnPTCPwrAct]
  sigCbnSolarLeft/1(CAN3_sigCbnSolarLeft) -> [CAN3_sigCbnSolarLeft]
  sigCbnSolarRight/1(CAN3_sigCbnSolarRight) -> [CAN3_sigCbnSolarRight]
  sigClmtCmprPwrAct/1(CAN3_sigClmtCmprPwrAct) -> [CAN3_sigClmtCmprPwrAct]
  sigClntTHvBattOut/1(CAN3_sigClntTHvBattOut) -> [CAN3_sigClntTHvBattOut]
  sigDfrstSt/1(CAN3_sigDfrstSt) -> [CAN3_sigDfrstSt]
  sigHvacSt/1(CAN3_sigHvacSt) -> [CAN3_sigHvacSt]
  sigRecircSt/1(CAN3_sigRecircSt) -> [CAN3_sigRecircSt]
  sigSetTempZon1St/1(CAN3_sigSetTempZon1St) -> [CAN3_sigSetTempZon1St]
  sigSetTempZon2St/1(CAN3_sigSetTempZon2St) -> [CAN3_sigSetTempZon2St]
  sigSetTempZon3St/1(CAN3_sigSetTempZon3St) -> [CAN3_sigSetTempZon3St]
  sigWindDirZon1St/1(CAN3_sigWindDirZon1St) -> [CAN3_sigWindDirZon1St]
  sigWindDirZon3St/1(CAN3_sigWindDirZon3St) -> [CAN3_sigWindDirZon3St]
  bus_selector/1 -> BatteryMode/1(BatteryMode)  "<VOUTP_BatteryMode_enum>"
  [BOUTP_outputs] -> bus_selector/1
  bus_selector1/1 -> CCUACLampSts/1(CCUACLampSts)  "<VOUTP_CCUACLampSts_flg>"
  [BOUTP_outputs] -> bus_selector1/1
  bus_selector2/1 -> CCUACMaxLampSts/1(CCUACMaxLampSts)  "<VOUTP_CCUACMaxLampSts_flg>"
  [BOUTP_outputs] -> bus_selector2/1
  bus_selector3/1 -> CCUAutoLampSts/1(CCUAutoLampSts)  "<VOUTP_CCUAutoLampSts_flg>"
  [BOUTP_outputs] -> bus_selector3/1
  Ground/1 -> CCUAutoMidLampSts/1(CCUAutoMidLampSts)
  Ground1/1 -> CCUDispalyRequest/1(CCUDispalyRequest)
  Ground2/1 -> CCUEcoSts/1(CCUEcoSts)
  Ground3/1 -> CCUFrtOnOffLampSts/1(CCUFrtOnOffLampSts)
  Ground4/1 -> CCUHEATMaxLampSts/1(CCUHEATMaxLampSts)
  Ground5/1 -> CCURrOnOffLampSts/1(CCURrOnOffLampSts)
  bus_selector4/1 -> CCUSyncLampSts/1(CCUSyncLampSts)  "<VOUTP_CCUSyncLampSts_flg>"
  [BOUTP_outputs] -> bus_selector4/1
  bus_selector5/1 -> CabinMode/1(CabinMode)  "<VOUTP_CabinMode_enum>"
  [BOUTP_outputs] -> bus_selector5/1
  bus_selector6/1 -> EDriveMode/1(EDriveMode)  "<VOUTP_EDriveMode_enum>"
  [BOUTP_outputs] -> bus_selector6/1
  bus_selector7/1 -> FDAGSCmd/1(FDAGSCmd)  "<VOUTP_FDAGSCmd_enum>"
  [BOUTP_outputs] -> bus_selector7/1
  bus_selector8/1 -> FDRecyAutoCmd/1(FDRecyAutoCmd)  "<VOUTP_FDRecyAutoCmd_enum>"
  [BOUTP_outputs] -> bus_selector8/1
  Ground6/1 -> FrCoolantflow/1(FrCoolantflow)
  Ground7/1 -> FrCoolanttemp/1(FrCoolanttemp)
  Ground8/1 -> HPThermalRecoveryReq/1(HPThermalRecoveryReq)
  Ground9/1 -> RrCoolantflow/1(RrCoolantflow)
  Ground10/1 -> RrCoolanttemp/1(RrCoolanttemp)
  bus_selector9/1 -> sigAirIntenZon1St/1(sigAirIntenZon1St)  "<VOUTP_sigAirIntenZon1St_enum>"
  [BOUTP_outputs] -> bus_selector9/1
  Ground11/1 -> sigAirIntenZon3St/1(sigAirIntenZon3St)
  bus_selector10/1 -> sigAmbAirT/1(sigAmbAirT)  "<VOUTP_sigAmbAirT_C>"
  [BOUTP_outputs] -> bus_selector10/1
  bus_selector11/1 -> sigCbnAirT/1(sigCbnAirT)  "<VOUTP_sigCbnAirT_C>"
  [BOUTP_outputs] -> bus_selector11/1
  Ground12/1 -> sigCbnPTCPwrAct/1(sigCbnPTCPwrAct)
  bus_selector12/1 -> sigCbnSolarLeft/1(sigCbnSolarLeft)  "<VOUTP_sigCbnSolarLeft_W>"
  [BOUTP_outputs] -> bus_selector12/1
  bus_selector13/1 -> sigCbnSolarRight/1(sigCbnSolarRight)  "<VOUTP_sigCbnSolarRight_W>"
  [BOUTP_outputs] -> bus_selector13/1
  Ground13/1 -> sigClmtCmprPwrAct/1(sigClmtCmprPwrAct)
  bus_selector14/1 -> sigClntTHvBattOut/1(sigClntTHvBattOut)  "<VOUTP_sigClntTHvBattOut_C>"
  [BOUTP_outputs] -> bus_selector14/1
  bus_selector15/1 -> sigDfrstSt/1(sigDfrstSt)  "<VOUTP_sigDfrstSt_flg>"
  [BOUTP_outputs] -> bus_selector15/1
  Ground14/1 -> sigHvacSt/1(sigHvacSt)
  bus_selector16/1 -> sigRecircSt/1(sigRecircSt)  "<VOUTP_sigRecircSt_flg>"
  [BOUTP_outputs] -> bus_selector16/1
  bus_selector17/1 -> sigSetTempZon1St/1(sigSetTempZon1St)  "<VOUTP_sigSetTempZon1St_C>"
  [BOUTP_outputs] -> bus_selector17/1
  bus_selector18/1 -> sigSetTempZon2St/1(sigSetTempZon2St)  "<VOUTP_sigSetTempZon2St_C>"
  [BOUTP_outputs] -> bus_selector18/1
  Ground15/1 -> sigSetTempZon3St/1(sigSetTempZon3St)
  bus_selector19/1 -> sigWindDirZon1St/1(sigWindDirZon1St)  "<VOUTP_sigWindDirZon1St_enum>"
  [BOUTP_outputs] -> bus_selector19/1
  Ground16/1 -> sigWindDirZon3St/1(sigWindDirZon3St)

== system halout/HAL_OUT/CAN3/FD3_THCM2_0x186 ==
  BSCP_outputs : Inport  OutDataTypeStr=Bus: BSCP_outputs
  BOUTP_outputs : Inport  Port=2  OutDataTypeStr=Bus: BOUTP_outputs
  ACSubMode : Subsystem
  APTCActFrRiPwr : Subsystem
  BatLoopActWtFlw : Subsystem
  CCUCbnPreACWkSts : Subsystem
  CCUCbnPreEstimdTi : Subsystem
  CCUCbnPreSts : Subsystem
  CCUHiVoltageReq : Subsystem
  CoolgFanActDuty : Subsystem
  DeiceModReq : Subsystem
  FDBlowerCmd : Subsystem
  FDCompCmd : Subsystem
  FDEWP1Cmd : Subsystem
  FDEWP2Cmd : Subsystem
  FDEWP3Cmd : Subsystem
  FDEXV1Cmd : Subsystem
  FDEXV2Cmd : Subsystem
  FDFWVCmd : Subsystem
  FDFrLeAPTCHeatPwrCmd : Subsystem
  FDFrRiAPTCHeatPwrCmd : Subsystem
  FDFrWPTCHeatPwrCmd : Subsystem
  FDRrAPTCHeatPwrCmd : Subsystem
  FDSOTXVCmd : Subsystem
  FDSOV1Cmd : Subsystem
  FDSOV2Cmd : Subsystem
  FDSOV3Cmd : Subsystem
  FDTWVCmd : Subsystem
  Ground{,1..6} (7 alike) : Ground
  bus_creator : BusCreator  Inputs=26  OutDataTypeStr=Bus: DT_CAN3_SG_FD3_THCM2  NonVirtualBus=on
  bus_selector : BusSelector  OutputSignals=VOUTP_ACSubMode_enum
  bus_selector1 : BusSelector  OutputSignals=VOUTP_CoolgFanActDuty_pct
  bus_selector10 : BusSelector  OutputSignals=VOUTP_FDFrLeAPTCHeatPwrCmd_W
  bus_selector11 : BusSelector  OutputSignals=VOUTP_FDFrRiAPTCHeatPwrCmd_W
  bus_selector12 : BusSelector  OutputSignals=VOUTP_FDFrWPTCHeatPwrCmd_W
  bus_selector13 : BusSelector  OutputSignals=VOUTP_FDRrAPTCHeatPwrCmd_W
  bus_selector14 : BusSelector  OutputSignals=VOUTP_FDSOTXVCmd_flg
  bus_selector15 : BusSelector  OutputSignals=VOUTP_FDSOV1Cmd_flg
  bus_selector16 : BusSelector  OutputSignals=VOUTP_FDSOV2Cmd_flg
  bus_selector17 : BusSelector  OutputSignals=VOUTP_FDSOV3Cmd_flg
  bus_selector18 : BusSelector  OutputSignals=VOUTP_FDTWVCmd_pct
  bus_selector2 : BusSelector  OutputSignals=VOUTP_FDBlowerCmd_pct
  bus_selector3 : BusSelector  OutputSignals=VOUTP_FDCompCmd_rpm
  bus_selector4 : BusSelector  OutputSignals=VOUTP_FDEWP1Cmd_enum
  bus_selector5 : BusSelector  OutputSignals=VOUTP_FDEWP2Cmd_enum
  bus_selector6 : BusSelector  OutputSignals=VOUTP_FDEWP3Cmd_enum
  bus_selector7 : BusSelector  OutputSignals=VOUTP_FDEXV1Cmd_step
  bus_selector8 : BusSelector  OutputSignals=VOUTP_FDEXV2Cmd_step
  bus_selector9 : BusSelector  OutputSignals=VOUTP_FDFWVCmd_flg
  FD3_THCM2 : Outport
  wires:
  BSCP_outputs/1 -> [BSCP_outputs]
  BOUTP_outputs/1 -> [BOUTP_outputs]
  [CAN3_ACSubMode] -> bus_creator/1  "CAN3_ACSubMode"
  [CAN3_APTC_ActFrRiPwr] -> bus_creator/2  "CAN3_APTC_ActFrRiPwr"
  [CAN3_BatLoopActWtFlw] -> bus_creator/3  "CAN3_BatLoopActWtFlw"
  [CAN3_CCU_CbnPreACWkSts] -> bus_creator/4  "CAN3_CCU_CbnPreACWkSts"
  [CAN3_CCU_CbnPreEstimdTi] -> bus_creator/5  "CAN3_CCU_CbnPreEstimdTi"
  [CAN3_CCU_CbnPreSts] -> bus_creator/6  "CAN3_CCU_CbnPreSts"
  [CAN3_CCU_HiVoltageReq] -> bus_creator/7  "CAN3_CCU_HiVoltageReq"
  [CAN3_CoolgFanActDuty] -> bus_creator/8  "CAN3_CoolgFanActDuty"
  [CAN3_DeiceModReq] -> bus_creator/9  "CAN3_DeiceModReq"
  [CAN3_FD_Blower_Cmd] -> bus_creator/10  "CAN3_FD_Blower_Cmd"
  [CAN3_FD_Comp_Cmd] -> bus_creator/11  "CAN3_FD_Comp_Cmd"
  [CAN3_FD_EWP1_Cmd] -> bus_creator/12  "CAN3_FD_EWP1_Cmd"
  [CAN3_FD_EWP2_Cmd] -> bus_creator/13  "CAN3_FD_EWP2_Cmd"
  [CAN3_FD_EWP3_Cmd] -> bus_creator/14  "CAN3_FD_EWP3_Cmd"
  [CAN3_FD_EXV1_Cmd] -> bus_creator/15  "CAN3_FD_EXV1_Cmd"
  [CAN3_FD_EXV2_Cmd] -> bus_creator/16  "CAN3_FD_EXV2_Cmd"
  [CAN3_FD_FWV_Cmd] -> bus_creator/17  "CAN3_FD_FWV_Cmd"
  [CAN3_FD_FrLeAPTCHeatPwr_Cmd] -> bus_creator/18  "CAN3_FD_FrLeAPTCHeatPwr_Cmd"
  [CAN3_FD_FrRiAPTCHeatPwr_Cmd] -> bus_creator/19  "CAN3_FD_FrRiAPTCHeatPwr_Cmd"
  [CAN3_FD_FrWPTCHeatPwr_Cmd] -> bus_creator/20  "CAN3_FD_FrWPTCHeatPwr_Cmd"
  [CAN3_FD_RrAPTCHeatPwr_Cmd] -> bus_creator/21  "CAN3_FD_RrAPTCHeatPwr_Cmd"
  [CAN3_FD_SOTXV_Cmd] -> bus_creator/22  "CAN3_FD_SOTXV_Cmd"
  [CAN3_FD_SOV1_Cmd] -> bus_creator/23  "CAN3_FD_SOV1_Cmd"
  [CAN3_FD_SOV2_Cmd] -> bus_creator/24  "CAN3_FD_SOV2_Cmd"
  [CAN3_FD_SOV3_Cmd] -> bus_creator/25  "CAN3_FD_SOV3_Cmd"
  [CAN3_FD_TWV_Cmd] -> bus_creator/26  "CAN3_FD_TWV_Cmd"
  bus_creator/1 -> FD3_THCM2/1
  ACSubMode/1(CAN3_ACSubMode) -> [CAN3_ACSubMode]
  APTCActFrRiPwr/1(CAN3_APTC_ActFrRiPwr) -> [CAN3_APTC_ActFrRiPwr]
  BatLoopActWtFlw/1(CAN3_BatLoopActWtFlw) -> [CAN3_BatLoopActWtFlw]
  CCUCbnPreACWkSts/1(CAN3_CCU_CbnPreACWkSts) -> [CAN3_CCU_CbnPreACWkSts]
  CCUCbnPreEstimdTi/1(CAN3_CCU_CbnPreEstimdTi) -> [CAN3_CCU_CbnPreEstimdTi]
  CCUCbnPreSts/1(CAN3_CCU_CbnPreSts) -> [CAN3_CCU_CbnPreSts]
  CCUHiVoltageReq/1(CAN3_CCU_HiVoltageReq) -> [CAN3_CCU_HiVoltageReq]
  CoolgFanActDuty/1(CAN3_CoolgFanActDuty) -> [CAN3_CoolgFanActDuty]
  DeiceModReq/1(CAN3_DeiceModReq) -> [CAN3_DeiceModReq]
  FDBlowerCmd/1(CAN3_FD_Blower_Cmd) -> [CAN3_FD_Blower_Cmd]
  FDCompCmd/1(CAN3_FD_Comp_Cmd) -> [CAN3_FD_Comp_Cmd]
  FDEWP1Cmd/1(CAN3_FD_EWP1_Cmd) -> [CAN3_FD_EWP1_Cmd]
  FDEWP2Cmd/1(CAN3_FD_EWP2_Cmd) -> [CAN3_FD_EWP2_Cmd]
  FDEWP3Cmd/1(CAN3_FD_EWP3_Cmd) -> [CAN3_FD_EWP3_Cmd]
  FDEXV1Cmd/1(CAN3_FD_EXV1_Cmd) -> [CAN3_FD_EXV1_Cmd]
  FDEXV2Cmd/1(CAN3_FD_EXV2_Cmd) -> [CAN3_FD_EXV2_Cmd]
  FDFWVCmd/1(CAN3_FD_FWV_Cmd) -> [CAN3_FD_FWV_Cmd]
  FDFrLeAPTCHeatPwrCmd/1(CAN3_FD_FrLeAPTCHeatPwr_Cmd) -> [CAN3_FD_FrLeAPTCHeatPwr_Cmd]
  FDFrRiAPTCHeatPwrCmd/1(CAN3_FD_FrRiAPTCHeatPwr_Cmd) -> [CAN3_FD_FrRiAPTCHeatPwr_Cmd]
  FDFrWPTCHeatPwrCmd/1(CAN3_FD_FrWPTCHeatPwr_Cmd) -> [CAN3_FD_FrWPTCHeatPwr_Cmd]
  FDRrAPTCHeatPwrCmd/1(CAN3_FD_RrAPTCHeatPwr_Cmd) -> [CAN3_FD_RrAPTCHeatPwr_Cmd]
  FDSOTXVCmd/1(CAN3_FD_SOTXV_Cmd) -> [CAN3_FD_SOTXV_Cmd]
  FDSOV1Cmd/1(CAN3_FD_SOV1_Cmd) -> [CAN3_FD_SOV1_Cmd]
  FDSOV2Cmd/1(CAN3_FD_SOV2_Cmd) -> [CAN3_FD_SOV2_Cmd]
  FDSOV3Cmd/1(CAN3_FD_SOV3_Cmd) -> [CAN3_FD_SOV3_Cmd]
  FDTWVCmd/1(CAN3_FD_TWV_Cmd) -> [CAN3_FD_TWV_Cmd]
  bus_selector/1 -> ACSubMode/1(ACSubMode)  "<VOUTP_ACSubMode_enum>"
  [BOUTP_outputs] -> bus_selector/1
  Ground/1 -> APTCActFrRiPwr/1(APTCActFrRiPwr)
  Ground1/1 -> BatLoopActWtFlw/1(BatLoopActWtFlw)
  Ground2/1 -> CCUCbnPreACWkSts/1(CCUCbnPreACWkSts)
  Ground3/1 -> CCUCbnPreEstimdTi/1(CCUCbnPreEstimdTi)
  Ground4/1 -> CCUCbnPreSts/1(CCUCbnPreSts)
  Ground5/1 -> CCUHiVoltageReq/1(CCUHiVoltageReq)
  bus_selector1/1 -> CoolgFanActDuty/1(CoolgFanActDuty)  "<VOUTP_CoolgFanActDuty_pct>"
  [BOUTP_outputs] -> bus_selector1/1
  Ground6/1 -> DeiceModReq/1(DeiceModReq)
  bus_selector2/1 -> FDBlowerCmd/1(FDBlowerCmd)  "<VOUTP_FDBlowerCmd_pct>"
  [BOUTP_outputs] -> bus_selector2/1
  bus_selector3/1 -> FDCompCmd/1(FDCompCmd)  "<VOUTP_FDCompCmd_rpm>"
  [BOUTP_outputs] -> bus_selector3/1
  bus_selector4/1 -> FDEWP1Cmd/1(FDEWP1Cmd)  "<VOUTP_FDEWP1Cmd_enum>"
  [BOUTP_outputs] -> bus_selector4/1
  bus_selector5/1 -> FDEWP2Cmd/1(FDEWP2Cmd)  "<VOUTP_FDEWP2Cmd_enum>"
  [BOUTP_outputs] -> bus_selector5/1
  bus_selector6/1 -> FDEWP3Cmd/1(FDEWP3Cmd)  "<VOUTP_FDEWP3Cmd_enum>"
  [BOUTP_outputs] -> bus_selector6/1
  bus_selector7/1 -> FDEXV1Cmd/1(FDEXV1Cmd)  "<VOUTP_FDEXV1Cmd_step>"
  [BOUTP_outputs] -> bus_selector7/1
  bus_selector8/1 -> FDEXV2Cmd/1(FDEXV2Cmd)  "<VOUTP_FDEXV2Cmd_step>"
  [BOUTP_outputs] -> bus_selector8/1
  bus_selector9/1 -> FDFWVCmd/1(FDFWVCmd)  "<VOUTP_FDFWVCmd_flg>"
  [BOUTP_outputs] -> bus_selector9/1
  bus_selector10/1 -> FDFrLeAPTCHeatPwrCmd/1(FDFrLeAPTCHeatPwrCmd)  "<VOUTP_FDFrLeAPTCHeatPwrCmd_W>"
  [BOUTP_outputs] -> bus_selector10/1
  bus_selector11/1 -> FDFrRiAPTCHeatPwrCmd/1(FDFrRiAPTCHeatPwrCmd)  "<VOUTP_FDFrRiAPTCHeatPwrCmd_W>"
  [BOUTP_outputs] -> bus_selector11/1
  bus_selector12/1 -> FDFrWPTCHeatPwrCmd/1(FDFrWPTCHeatPwrCmd)  "<VOUTP_FDFrWPTCHeatPwrCmd_W>"
  [BOUTP_outputs] -> bus_selector12/1
  bus_selector13/1 -> FDRrAPTCHeatPwrCmd/1(FDRrAPTCHeatPwrCmd)  "<VOUTP_FDRrAPTCHeatPwrCmd_W>"
  [BOUTP_outputs] -> bus_selector13/1
  bus_selector14/1 -> FDSOTXVCmd/1(FDSOTXVCmd)  "<VOUTP_FDSOTXVCmd_flg>"
  [BOUTP_outputs] -> bus_selector14/1
  bus_selector15/1 -> FDSOV1Cmd/1(FDSOV1Cmd)  "<VOUTP_FDSOV1Cmd_flg>"
  [BOUTP_outputs] -> bus_selector15/1
  bus_selector16/1 -> FDSOV2Cmd/1(FDSOV2Cmd)  "<VOUTP_FDSOV2Cmd_flg>"
  [BOUTP_outputs] -> bus_selector16/1
  bus_selector17/1 -> FDSOV3Cmd/1(FDSOV3Cmd)  "<VOUTP_FDSOV3Cmd_flg>"
  [BOUTP_outputs] -> bus_selector17/1
  bus_selector18/1 -> FDTWVCmd/1(FDTWVCmd)  "<VOUTP_FDTWVCmd_pct>"
  [BOUTP_outputs] -> bus_selector18/1

== system halout/HAL_OUT/CAN3/FD3_V2L1_0x374 ==
  BSCP_outputs : Inport  OutDataTypeStr=Bus: BSCP_outputs
  BOUTP_outputs : Inport  Port=2  OutDataTypeStr=Bus: BOUTP_outputs
  FDCV2LOBCExtrV2LCmd : Subsystem
  FDCV2LOBCIntrV2LCmd : Subsystem
  Ground : Ground
  ReqOBCV2LEna : Subsystem
  ReqV2LIVIPopup : Subsystem
  ReqV2LSwOn : Subsystem
  bus_creator : BusCreator  Inputs=5  OutDataTypeStr=Bus: DT_CAN3_SG_FD3_V2L1  NonVirtualBus=on
  bus_selector : BusSelector  OutputSignals=VOUTP_ReqOBCExtrV2LEna_enum
  bus_selector1 : BusSelector  OutputSignals=VOUTP_ReqOBCIntrV2LEna_enum
  bus_selector2 : BusSelector  OutputSignals=VOUTP_ReqOBCV2LEna_enum
  bus_selector3 : BusSelector  OutputSignals=VOUTP_ReqV2LIVIPopup_enum
  FD3_V2L1 : Outport
  wires:
  BSCP_outputs/1 -> [BSCP_outputs]
  BOUTP_outputs/1 -> [BOUTP_outputs]
  [CAN3_FDC_V2L_OBCExtrV2L_Cmd] -> bus_creator/1  "CAN3_FDC_V2L_OBCExtrV2L_Cmd"
  [CAN3_FDC_V2L_OBCIntrV2L_Cmd] -> bus_creator/2  "CAN3_FDC_V2L_OBCIntrV2L_Cmd"
  [CAN3_Req_OBCV2LEna] -> bus_creator/3  "CAN3_Req_OBCV2LEna"
  [CAN3_Req_V2LSwOn] -> bus_creator/4  "CAN3_Req_V2LSwOn"
  [CAN3_Req_V2L_IVI_Popup] -> bus_creator/5  "CAN3_Req_V2L_IVI_Popup"
  bus_creator/1 -> FD3_V2L1/1
  FDCV2LOBCExtrV2LCmd/1(CAN3_FDC_V2L_OBCExtrV2L_Cmd) -> [CAN3_FDC_V2L_OBCExtrV2L_Cmd]
  FDCV2LOBCIntrV2LCmd/1(CAN3_FDC_V2L_OBCIntrV2L_Cmd) -> [CAN3_FDC_V2L_OBCIntrV2L_Cmd]
  ReqOBCV2LEna/1(CAN3_Req_OBCV2LEna) -> [CAN3_Req_OBCV2LEna]
  ReqV2LSwOn/1(CAN3_Req_V2LSwOn) -> [CAN3_Req_V2LSwOn]
  ReqV2LIVIPopup/1(CAN3_Req_V2L_IVI_Popup) -> [CAN3_Req_V2L_IVI_Popup]
  bus_selector/1 -> FDCV2LOBCExtrV2LCmd/1(FDCV2LOBCExtrV2LCmd)  "<VOUTP_ReqOBCExtrV2LEna_enum>"
  [BOUTP_outputs] -> bus_selector/1
  bus_selector1/1 -> FDCV2LOBCIntrV2LCmd/1(FDCV2LOBCIntrV2LCmd)  "<VOUTP_ReqOBCIntrV2LEna_enum>"
  [BOUTP_outputs] -> bus_selector1/1
  bus_selector2/1 -> ReqOBCV2LEna/1(ReqOBCV2LEna)  "<VOUTP_ReqOBCV2LEna_enum>"
  [BOUTP_outputs] -> bus_selector2/1
  Ground/1 -> ReqV2LSwOn/1(ReqV2LSwOn)
  bus_selector3/1 -> ReqV2LIVIPopup/1(ReqV2LIVIPopup)  "<VOUTP_ReqV2LIVIPopup_enum>"
  [BOUTP_outputs] -> bus_selector3/1
